simulink model "LaunchFromCanister"  (R2022a)
settings: Solver=FixedStepAuto  StartTime=0.0  StopTime=2  FixedStep=0.001  RelTol=1e-3
libraries: robotlib x17, robotgazebolib x9, slpidlib x1, simulink x1
settings Model: Creator=abiyyumufti  LastModifiedBy=amani

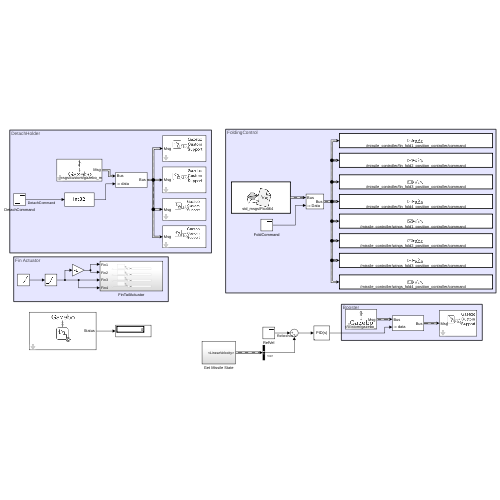
[thumbnail: Simulink's stored preview of the top-level diagram]
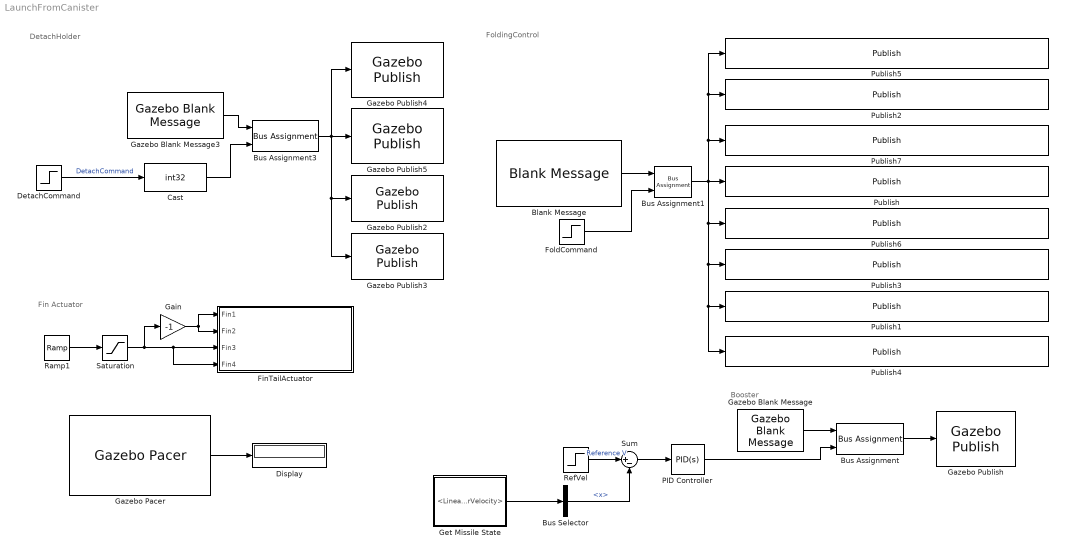
== system LaunchFromCanister ==
  note: FoldingControl
  note: DetachHolder
  note: Fin Actuator
  note: Booster
  Blank Message : robotlib/Blank Message  messageClass=Message  entityType=std_msgs/Float64  messageType=std_msgs/Float64  SampleTime=inf  legacyBusStruct=off
  Bus Assignment : BusAssignment  AssignedSignals=data
  Bus Assignment1 : BusAssignment  AssignedSignals=Data
  Bus Assignment3 : BusAssignment  AssignedSignals=data
  Bus Selector : BusSelector  OutputSignals=LinearVelocity.x
  Cast : DataTypeConversion  OutDataTypeStr=int32  SaturateOnIntegerOverflow=off  RndMeth=Floor
  DetachCommand : Step  Time=0.15  SampleTime=0
  Display : Display
  FinTailActuator : Subsystem
  FoldCommand : Step  Time=0.3  After=deg2rad(123)  SampleTime=0
  Gain : Gain  Gain=-1
  Gazebo Blank Message : robotgazebolib/Gazebo Blank Message  msgType=gazebo_msgs/custom/gazebo_msgs/Double  sampleTime=0.001  busName='Gazebo_SL_Bus_gazebo_msgs_custom_gazebo_msgs_Double'
      settings: SourceProductBaseCode=RO
  Gazebo Blank Message3 : robotgazebolib/Gazebo Blank Message  msgType=gazebo_msgs/custom/gazebo_msgs/Int  sampleTime=0.001  busName='Gazebo_SL_Bus_gazebo_msgs_custom_gazebo_msgs_Int'
      settings: SourceProductBaseCode=RO
  Gazebo Pacer : robotgazebolib/Gazebo Pacer  ResetBehavior=Reset Gazebo simulation time and scene  SampleTime=0.001
      settings: SourceProductBaseCode=RO
  Gazebo Publish : robotgazebolib/Gazebo Publish  topicSource=Specify your own  topic=/gazebo/my_world/booster_force  messageType=gazebo_msgs/custom/gazebo_msgs/Double  sampleTime=0.001
      settings: SourceProductBaseCode=RO
  Gazebo Publish2 : robotgazebolib/Gazebo Publish  topicSource=Specify your own  topic=/gazebo/my_world/holder1_detach  messageType=gazebo_msgs/custom/gazebo_msgs/Int  sampleTime=0.001
      settings: SourceProductBaseCode=RO
  Gazebo Publish3 : robotgazebolib/Gazebo Publish  topicSource=Specify your own  topic=/gazebo/my_world/holder2_detach  messageType=gazebo_msgs/custom/gazebo_msgs/Int  sampleTime=0.001
      settings: SourceProductBaseCode=RO
  Gazebo Publish4 : robotgazebolib/Gazebo Publish  topicSource=Specify your own  topic=/gazebo/my_world/holder3_detach  messageType=gazebo_msgs/custom/gazebo_msgs/Int  sampleTime=0.001
      settings: SourceProductBaseCode=RO
  Gazebo Publish5 : robotgazebolib/Gazebo Publish  topicSource=Specify your own  topic=/gazebo/my_world/holder4_detach  messageType=gazebo_msgs/custom/gazebo_msgs/Int  sampleTime=0.001
      settings: SourceProductBaseCode=RO
  Get Missile State : Subsystem
  PID Controller : slpidlib/PID Controller  Controller=PID  Form=Parallel  TimeDomain=Continuous-time  UseExternalTs=off  SampleTime=-1  IntegratorMethod=Forward Euler  FilterMethod=Forward Euler  ControllerParametersSource=internal  P=1000  I=0  UseKiTs=off  D=15  N=100  UseFilter=on  TunerSelectOption=Transfer Function Based (PID Tuner App)  InitialConditionSource=internal  InitialConditionForIntegrator=0  InitialConditionForFilter=0  DifferentiatorICPrevScaledInput=0  ExternalReset=none  TrackingMode=off  Kt=1  LimitOutput=off  SatLimitsSource=internal  UpperSaturationLimit=inf  LowerSaturationLimit=-inf  LinearizeAsGain=on  AntiWindupMode=none  Kb=1  POutMin=[]  POutMax=[]  IOutMin=[]  IOutMax=[]  DOutMin=[]  DOutMax=[]  NOutMin=[]  NOutMax=[]  SumOutMin=[]  SumOutMax=[]  SaturationOutMin=[]  SaturationOutMax=[]  PParamMin=[]  PParamMax=[]  IParamMin=[]  IParamMax=[]  DParamMin=[]  DParamMax=[]  NParamMin=[]  NParamMax=[]  KbParamMin=[]  KbParamMax=[]  KtParamMin=[]  KtParamMax=[]  KbOutMin=[]  KbOutMax=[]  KtOutMin=[]  KtOutMax=[]  IntegratorOutMin=[]  IntegratorOutMax=[]  FilterOutMin=[]  FilterOutMax=[]  SumI1OutMin=[]  SumI1OutMax=[]  SumI2OutMin=[]  SumI2OutMax=[]  SumI3OutMin=[]  SumI3OutMax=[]  SumI4OutMin=[]  SumI4OutMax=[]  SumDOutMin=[]  SumDOutMax=[]  DifferentiatorOutMin=[]  DifferentiatorOutMax=[]  FilterDiffOutCoefMin=[]  FilterDiffOutCoefMax=[]  ReciprocalOutMin=[]  ReciprocalOutMax=[]  SumDenOutMin=[]  SumDenOutMax=[]  SumNumOutMin=[]  SumNumOutMax=[]  DivideOutMin=[]  DivideOutMax=[]  UdiffTsProdOutMin=[]  UdiffTsProdOutMax=[]  NTsProdOutMin=[]  NTsProdOutMax=[]  UintegralTsProdOutMin=[]  UintegralTsProdOutMax=[]  UngainTsProdOutMin=[]  UngainTsProdOutMax=[]  IntegratorContinuousStateAttributes=''  IntegratorStateMustResolveToSignalObject=off  IntegratorRTWStateStorageClass=Auto  FilterContinuousStateAttributes=''  FilterStateMustResolveToSignalObject=off  FilterRTWStateStorageClass=Auto  ParallelPVariant=InternalParameters  IdealPVariant=Disabled  IVariant=InternalParameters  DVariant=InternalParameters  IntegratorVariant=Continuous  SatVariant=Disabled  AWVariant=Passthrough  PCopyVariant=Disabled  TRVariant=Disabled  FdbkBlocksVariant=Forward  IdealPFdbkVariant=Disabled  SatFdbkVariant=Disabled  DerivativeFilterVariant=ContFilter  NVariant=InternalParameters  NCopyVariant=Disabled  FilterICVariant=InternalICsFilter  IntegratorICVariant=InternalICs  ExternalResetVariant=Disabled  TRSumVariant=Passthrough  SumFdbkVariant=Disabled  SumVariant=Sum_PID  TsampFilterVariant=InternalTs  TsampNgainVariant=Passthrough  TsampIntegralVariant=Passthrough  ExternalSaturationOutDataTypeStr=Inherit: Same as second input  aMode=0
  Publish : robotlib/Publish  topicSource=Select from ROS network  topic=/missile_controller/fin_fold4_position_controller/command  messageType=std_msgs/Float64  legacyBusStruct=off  messageQueueLength=1
  Publish1 : robotlib/Publish  topicSource=Select from ROS network  topic=/missile_controller/wings_fold3_position_controller/command  messageType=std_msgs/Float64  legacyBusStruct=off  messageQueueLength=1
  Publish2 : robotlib/Publish  topicSource=Select from ROS network  topic=/missile_controller/fin_fold2_position_controller/command  messageType=std_msgs/Float64  legacyBusStruct=off  messageQueueLength=1
  Publish3 : robotlib/Publish  topicSource=Select from ROS network  topic=/missile_controller/wings_fold2_position_controller/command  messageType=std_msgs/Float64  legacyBusStruct=off  messageQueueLength=1
  Publish4 : robotlib/Publish  topicSource=Select from ROS network  topic=/missile_controller/wings_fold4_position_controller/command  messageType=std_msgs/Float64  legacyBusStruct=off  messageQueueLength=1
  Publish5 : robotlib/Publish  topicSource=Select from ROS network  topic=/missile_controller/fin_fold1_position_controller/command  messageType=std_msgs/Float64  legacyBusStruct=off  messageQueueLength=1
  Publish6 : robotlib/Publish  topicSource=Select from ROS network  topic=/missile_controller/wings_fold1_position_controller/command  messageType=std_msgs/Float64  legacyBusStruct=off  messageQueueLength=1
  Publish7 : robotlib/Publish  topicSource=Select from ROS network  topic=/missile_controller/fin_fold3_position_controller/command  messageType=std_msgs/Float64  legacyBusStruct=off  messageQueueLength=1
  Ramp1 : simulink/Sources/Ramp  slope=-deg2rad(20)/5  start=10  InitialOutput=0
  RefVel : Step  Time=1e-3  After=250  SampleTime=0
  Saturation : Saturate  UpperLimit=deg2rad(10)  LowerLimit=-deg2rad(10)
  Sum : Sum  Inputs=|+-
  wires:
  Gazebo Blank Message/1 -> Bus Assignment/1
  Blank Message/1 -> Bus Assignment1/1
  FoldCommand/1 -> Bus Assignment1/2
  RefVel/1 -> Sum/1  "Reference V"
  Saturation/1 -> FinTailActuator/4(Fin4), FinTailActuator/3(Fin3), Gain/1
  Bus Assignment/1 -> Gazebo Publish/1
  Sum/1 -> PID Controller/1
  Get Missile State/1(<LinearVelocity>) -> Bus Selector/1
  Gazebo Pacer/1 -> Display/1
  DetachCommand/1 -> Cast/1  "DetachCommand"
  Bus Selector/1 -> Sum/2  "<x>"
  Ramp1/1 -> Saturation/1
  Bus Assignment1/1 -> Publish4/1, Publish1/1, Publish3/1, Publish6/1, Publish5/1, Publish2/1, Publish7/1, Publish/1
  Gain/1 -> FinTailActuator/2(Fin2), FinTailActuator/1(Fin1)
  Gazebo Blank Message3/1 -> Bus Assignment3/1
  Cast/1 -> Bus Assignment3/2
  Bus Assignment3/1 -> Gazebo Publish3/1, Gazebo Publish2/1, Gazebo Publish4/1, Gazebo Publish5/1
  PID Controller/1 -> Bus Assignment/2

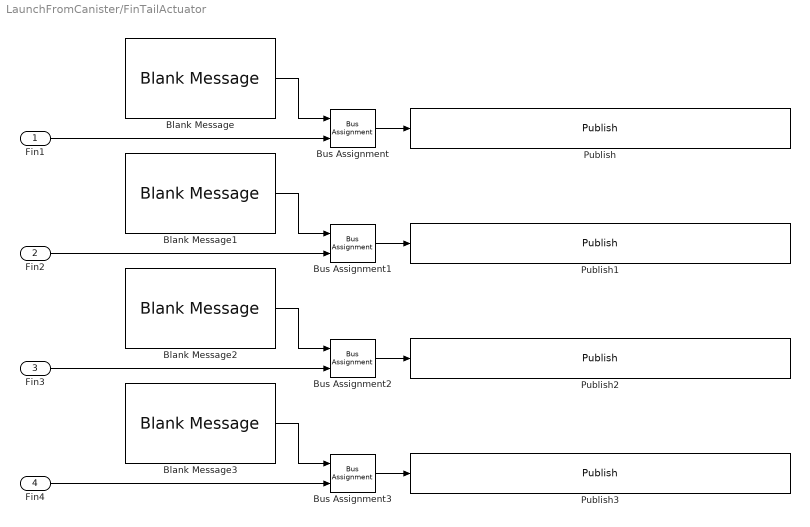
== system LaunchFromCanister/FinTailActuator ==
  Fin1 : Inport
  Fin2 : Inport  Port=2
  Fin3 : Inport  Port=3
  Fin4 : Inport  Port=4
  Blank Message{,1..3} (4 alike) : robotlib/Blank Message  messageClass=Message  entityType=std_msgs/Float64  messageType=std_msgs/Float64  SampleTime=inf  legacyBusStruct=off
  Bus Assignment{,1..3} (4 alike) : BusAssignment  AssignedSignals=Data
  Publish : robotlib/Publish  topicSource=Select from ROS network  topic=/missile_controller/fins_rev1_position_controller/command  messageType=std_msgs/Float64  legacyBusStruct=off  messageQueueLength=1
  Publish1 : robotlib/Publish  topicSource=Select from ROS network  topic=/missile_controller/fins_rev2_position_controller/command  messageType=std_msgs/Float64  legacyBusStruct=off  messageQueueLength=1
  Publish2 : robotlib/Publish  topicSource=Select from ROS network  topic=/missile_controller/fins_rev3_position_controller/command  messageType=std_msgs/Float64  legacyBusStruct=off  messageQueueLength=1
  Publish3 : robotlib/Publish  topicSource=Select from ROS network  topic=/missile_controller/fins_rev4_position_controller/command  messageType=std_msgs/Float64  legacyBusStruct=off  messageQueueLength=1
  wires:
  Fin1/1 -> Bus Assignment/2
  Bus Assignment3/1 -> Publish3/1
  Blank Message/1 -> Bus Assignment/1
  Fin4/1 -> Bus Assignment3/2
  Bus Assignment1/1 -> Publish1/1
  Blank Message3/1 -> Bus Assignment3/1
  Blank Message2/1 -> Bus Assignment2/1
  Bus Assignment/1 -> Publish/1
  Blank Message1/1 -> Bus Assignment1/1
  Bus Assignment2/1 -> Publish2/1
  Fin2/1 -> Bus Assignment1/2
  Fin3/1 -> Bus Assignment2/2

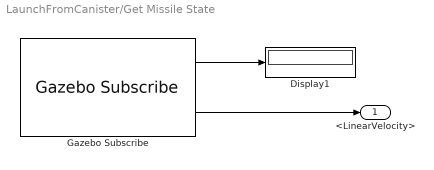
== system LaunchFromCanister/Get Missile State ==
  Display1 : Display
  Gazebo Subscribe : robotgazebolib/Gazebo Subscribe  topicSource=From Gazebo  topic=/gazebo/my_world/DynamicState  messageType=gazebo_msgs/custom/ssm_msgs_msgs/DynamicState  sampleTime=0.001
      settings: SourceProductBaseCode=RO
  <LinearVelocity> : Outport
  wires:
  Gazebo Subscribe/1 -> Display1/1
  Gazebo Subscribe/2 -> <LinearVelocity>/1
